simulink model "Controller"  (R2019b)
settings: Solver=ode4  StartTime=0.0  StopTime=5  FixedStep=0.01  RelTol=1e-3  EnableMultiTasking=on
values from neighbouring files (symbols this model uses):
  Go = 1/ bode(G_hf*P*G_L,wc)    [LoopShaping_TP.m]
  m = 0.5    [LCS_freq.m]    (also in LoopShaping_TP.m = 2)
  w_hf = 300    [LoopShaping_TP.m]
  w_p = wc / tan(alpha)    [LoopShaping_TP.m]
  w_z = wc* tan(alpha)    [LoopShaping_TP.m]
settings Model: Creator=Thomas  LastModifiedBy=Ivan
settings DataIOCC: LimitDataPoints=on  SaveFormat=Array  ReturnWorkspaceOutputs=off
settings OptimizationCC: LifeSpan=inf
settings DebuggingCC: SolverPrmCheckMsg=warning  SFUnexpectedBacktrackingDiag=warning  SFNoUnconditionalDefaultTransitionDiag=warning  SFExecutionAtInitializationDiag=none  ArithmeticOperatorsInVariantConditions=warning
settings HardwareCC: ProdBitPerPointer=32  ProdBitPerSizeT=32  ProdBitPerPtrDiffT=32  ProdLargestAtomicFloat=None  ProdIntDivRoundTo=Undefined  ProdEndianess=Unspecified  ProdWordSize=32  ProdHWDeviceType=32-bit Generic
settings ModelReferenceCC: PropagateSignalLabelsOutOfModel=off
settings SFSimCC: SimUseLocalCustomCode=off  CustomCodeUndefinedFunction=UseInterfaceOnly
settings RTWCC: RTWUseLocalCustomCode=off
settings CodeAppCC: StateflowObjectComments=on
settings GRTTargetCC: TargetLangStandard=C89/C90 (ANSI)  GeneratePreprocessorConditionals=Disable all
settings ConfigComp: CovMetricSettings=dw  CovHtmlReporting=on  CovSaveCumulativeToWorkspaceVar=on  CovSaveSingleToWorkspaceVar=on  CovExternalEMLEnable=off  CovSFcnEnable=off

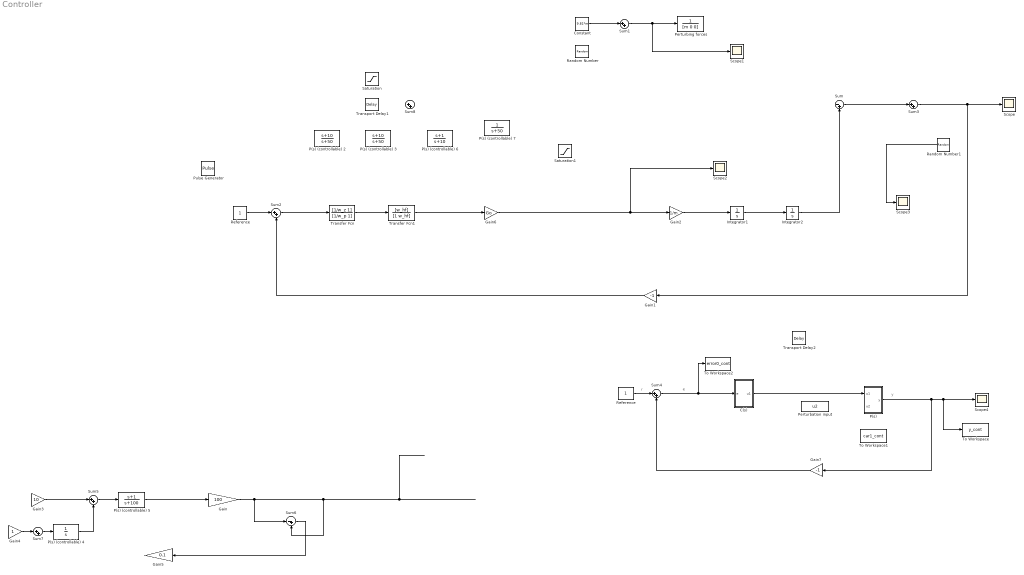
== system Controller ==
  note: e
  note: r
  note: y
  C(s) : Subsystem
  Constant : Constant  Value=9.81*m
  Gain : Gain  Gain=100
  Gain1 : Gain  Gain=-1
  Gain2 : Gain  Gain=1/m
  Gain3 : Gain  Gain=10
  Gain4 : Gain
  Gain5 : Gain  Gain=0.1
  Gain6 : Gain  Gain=Go
  Gain7 : Gain  Gain=-1
  Integrator1 : Integrator
  Integrator2 : Integrator
  P(s) : Subsystem
  P(s) (controllable) 2 : TransferFcn  Numerator=[1 10]  Denominator=[1 50]
  P(s) (controllable) 3 : TransferFcn  Numerator=[1 10]  Denominator=[1 50]
  P(s) (controllable) 4 : TransferFcn  Denominator=[1 0]
  P(s) (controllable) 5 : TransferFcn  Numerator=[1 1]  Denominator=[1 100]
  P(s) (controllable) 6 : TransferFcn  Numerator=[1 1]  Denominator=[1 10]
  P(s) (controllable) 7 : TransferFcn  Denominator=[1 50]
  Perturbation input : FromWorkspace  VariableName=u2  SampleTime=0
  "Perturbing forces " : TransferFcn  Denominator=[m 0 0]
  Pulse Generator : DiscretePulseGenerator  PulseType=Time based  Amplitude=0.5  Period=5  PulseWidth=50
  Random Number : RandomNumber  Seed=3  SampleTime=0.01
  Random Number1 : RandomNumber  Variance=0.0001  Seed=3  SampleTime=0.01
  Reference : Constant
  "Reference " : Constant
  Saturation : Saturate
  Saturation1 : Saturate  UpperLimit=10  LowerLimit=-10
  Scope{,1..4} (5 alike) : Scope
  Sum : Sum  Inputs=|-+
  Sum{1..5,7..8} (7 alike) : Sum  Inputs=|++
  Sum6 : Sum  Inputs=|-+
  To Workspace : ToWorkspace  VariableName=y_cont  SaveFormat=Timeseries  SampleTime=-1
  To Workspace1 : ToWorkspace  VariableName=car1_cont  SaveFormat=Timeseries  SampleTime=-1
  To Workspace2 : ToWorkspace  VariableName=error0_cont  SaveFormat=Timeseries  SampleTime=-1
  Transfer Fcn : TransferFcn  Numerator=[1/w_z 1]  Denominator=[1/w_p 1]
  Transfer Fcn1 : TransferFcn  Numerator=[w_hf]  Denominator=[1 w_hf]
  Transport Delay1 : TransportDelay
  Transport Delay2 : TransportDelay  DelayTime=0.05
  wires:
  Constant/1 -> Sum1/1
  Integrator1/1 -> Integrator2/1
  Sum1/1 -> Scope1/1, "Perturbing forces "/1
  Gain1/1 -> Sum2/2
  Sum/1 -> Sum3/1
  ? -> Gain4/1, Gain3/1
  Sum5/1 -> P(s) (controllable) 5/1
  P(s) (controllable) 4/1 -> Sum5/2
  Sum6/1 -> Gain5/1
  P(s) (controllable) 5/1 -> Gain/1
  Gain4/1 -> Sum7/1
  Sum7/1 -> P(s) (controllable) 4/1
  Gain3/1 -> Sum5/1
  Gain/1 -> Sum6/2, Sum6/1
  Sum2/1 -> Transfer Fcn/1
  Gain6/1 -> Gain2/1, Scope2/1
  Random Number1/1 -> Scope3/1
  Sum3/1 -> Gain1/1, Scope/1
  "Reference "/1 -> Sum2/1
  Transfer Fcn1/1 -> Gain6/1
  Transfer Fcn/1 -> Transfer Fcn1/1
  Integrator2/1 -> Sum/2
  Gain2/1 -> Integrator1/1
  Gain7/1 -> Sum4/2
  Reference/1 -> Sum4/1
  P(s)/1(y) -> Gain7/1, To Workspace/1, Scope4/1
  C(s)/1(u1) -> P(s)/1(u1)
  Sum4/1 -> To Workspace2/1, C(s)/1(e)

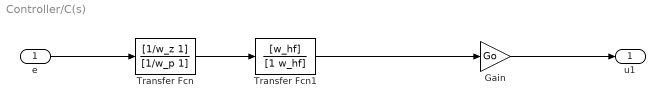
== system Controller/C(s) ==
  e : Inport
  Gain : Gain  Gain=Go
  Transfer Fcn : TransferFcn  Numerator=[1/w_z 1]  Denominator=[1/w_p 1]
  Transfer Fcn1 : TransferFcn  Numerator=[w_hf]  Denominator=[1 w_hf]
  u1 : Outport
  wires:
  e/1 -> Transfer Fcn/1
  Transfer Fcn/1 -> Transfer Fcn1/1
  Gain/1 -> u1/1
  Transfer Fcn1/1 -> Gain/1

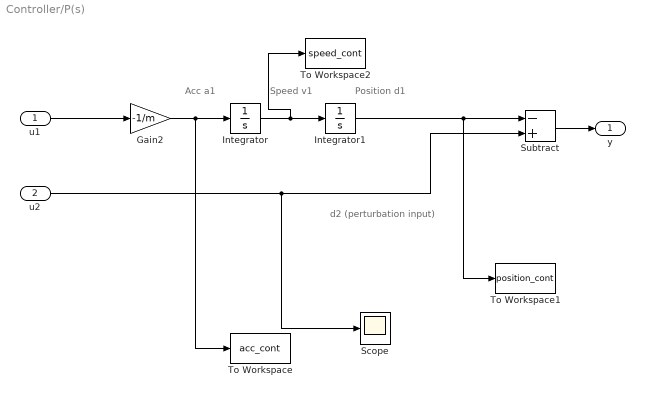
== system Controller/P(s) ==
  note: d2 (perturbation input)
  note: Position d1
  note: Speed v1
  note: Acc a1
  u1 : Inport
  u2 : Inport  Port=2
  Gain2 : Gain  Gain=-1/m
  Integrator : Integrator
  Integrator1 : Integrator
  Scope : Scope
  Subtract : Sum  Inputs=-+
  To Workspace : ToWorkspace  VariableName=acc_cont  SaveFormat=Timeseries  SampleTime=-1
  To Workspace1 : ToWorkspace  VariableName=position_cont  SaveFormat=Timeseries  SampleTime=-1
  To Workspace2 : ToWorkspace  VariableName=speed_cont  SaveFormat=Timeseries  SampleTime=-1
  y : Outport
  wires:
  u1/1 -> Gain2/1
  Subtract/1 -> y/1
  u2/1 -> Scope/1, Subtract/2
  Gain2/1 -> To Workspace/1, Integrator/1
  Integrator/1 -> To Workspace2/1, Integrator1/1
  Integrator1/1 -> To Workspace1/1, Subtract/1
